simulink library "utils_lib"  (R2020b)
settings: Solver=VariableStepAuto  StartTime=0.0  StopTime=10.0  RelTol=1e-3
undefined symbols (not defined in the file): encoderALeadsB, encoderCountPerRevolution
settings Model: Creator=promero  LastModifiedBy=manuel.fedou

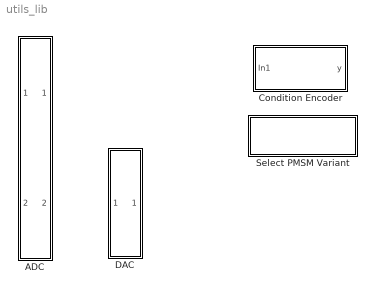
== system utils_lib ==
  ADC : Subsystem
      mask Display: disp('ADC')
  Condition Encoder : Subsystem  mask(Speedgoat Encoder Counter){cntsPerRevolution=encoderCountPerRevolution, positiveDirection=encoderALeadsB}
      mask prompts: cntsPerRevolution "Counts per revolution"; positiveDirection "A leads B?"
      mask help: Configures the direction and positive range of the counter value returned by the Speedgoat IO313 QAD Read block.
      mask init:
      | if positiveDirection == 1
      |     strPositiveDirection = 'A Leads B';
      | else
      |     strPositiveDirection = 'B Leads A';
      | end
      mask Display: fprintf(['Encoder\nPositive Direction:\n' strPositiveDirection]);
  DAC : Subsystem
      mask Display: disp('DAC')
  Select PMSM Variant : Subsystem  mask{pmsmVariant=PTBS}
      mask prompts: pmsmVariant "PMSM model variant:"
      mask TypeOptions pmsmVariant: MCB | Simscape | PTBS
      mask Callback pmsmVariant: Simulink.VariantConfigurationData.validateModel('PMSM_Plant_Model',[get_param(gcb,'pmsmVariant'),'_PMSM']);
      mask Display: fprintf('PMSM variant active:\n%s',pmsmVariant);

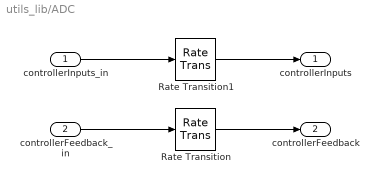
== system utils_lib/ADC ==
  controllerInputs_in : Inport
  controllerFeedback_in : Inport  Port=2
  Rate Transition : RateTransition  Integrity=off  Deterministic=off
  Rate Transition1 : RateTransition  Integrity=off
  controllerInputs : Outport  VectorParamsAs1DForOutWhenUnconnected=off
  controllerFeedback : Outport  Port=2  VectorParamsAs1DForOutWhenUnconnected=off
  wires:
  controllerFeedback_in/1 -> Rate Transition/1
  Rate Transition/1 -> controllerFeedback/1
  Rate Transition1/1 -> controllerInputs/1
  controllerInputs_in/1 -> Rate Transition1/1

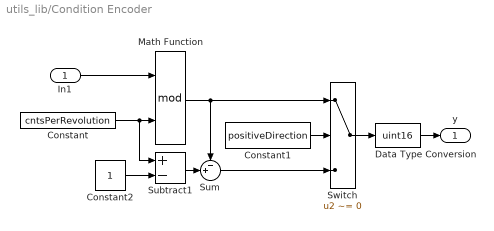
== system utils_lib/Condition Encoder ==
  In1 : Inport
  Constant : Constant  Value=cntsPerRevolution  OutDataTypeStr=Inherit: Inherit via back propagation
  Constant1 : Constant  Value=positiveDirection
  Constant2 : Constant  OutDataTypeStr=Inherit: Inherit via back propagation
  Data Type Conversion : DataTypeConversion  OutDataTypeStr=uint16
  Math Function : Math  Operator=mod  SignedPower=on  SaturateOnIntegerOverflow=on
  Subtract1 : Sum  Inputs=+-
  Sum : Sum  Inputs=-+|
  Switch : Switch  Criteria=u2 ~= 0
  y : Outport  VectorParamsAs1DForOutWhenUnconnected=off
  wires:
  Subtract1/1 -> Sum/2
  Constant2/1 -> Subtract1/2
  Constant/1 -> Math Function/2, Subtract1/1
  Sum/1 -> Switch/3
  Constant1/1 -> Switch/2
  Math Function/1 -> Switch/1, Sum/1
  In1/1 -> Math Function/1
  Switch/1 -> Data Type Conversion/1
  Data Type Conversion/1 -> y/1

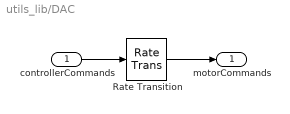
== system utils_lib/DAC ==
  controllerCommands : Inport
  Rate Transition : RateTransition  Integrity=off  Deterministic=off
  motorCommands : Outport
  wires:
  Rate Transition/1 -> motorCommands/1
  controllerCommands/1 -> Rate Transition/1

== system utils_lib/Select PMSM Variant ==
